simulink model "euler_equation"  (R2021b)
settings: Solver=VariableStepAuto  StartTime=0.0  StopTime=10.0  RelTol=1e-3
values from neighbouring files (symbols this model uses):
  J = [Ixx 0 0; 0 Iyy 0; 0 0 Izz]    [lab3_task1.m]    (also in lab3_task2.m; lab3_task3.m)
  Jinv = inv(J)    [lab3_task1.m]    (also in lab3_task2.m; lab3_task3.m)
  w0 = [0.45 0.52 0.55]'    [lab3_task1.m]    (also in lab3_task2.m; lab3_task3.m = w0_matrix(3,:)')
libraries: matrix_library x1
settings Model: Creator=samuz  LastModifiedBy=samuz

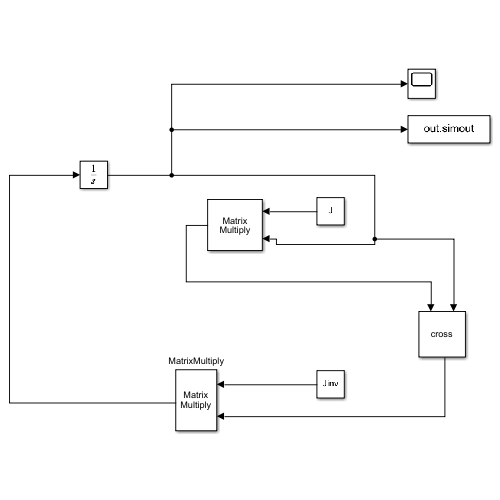
[thumbnail: Simulink's stored preview of the top-level diagram]
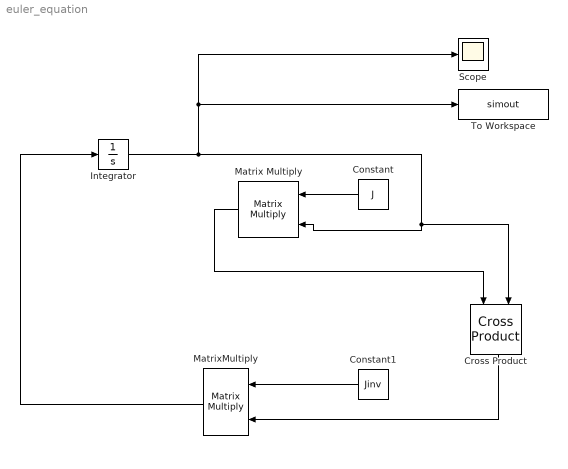
== system euler_equation ==
  Constant : Constant  Value=J
  Constant1 : Constant  Value=Jinv
  Cross Product : matrix_library/Cross Product
      settings: SourceProductBaseCode=SL
  Integrator : Integrator  InitialCondition=w0
  Matrix Multiply : Product  Multiplication=Matrix(*)
  MatrixMultiply : Product  Multiplication=Matrix(*)
  Scope : Scope
  To Workspace : ToWorkspace  VariableName=simout  SampleTime=-1
  wires:
  Matrix Multiply/1 -> Cross Product/1
  Cross Product/1 -> MatrixMultiply/2
  Integrator/1 -> Scope/1, To Workspace/1, Cross Product/2, Matrix Multiply/2
  Constant1/1 -> MatrixMultiply/1
  MatrixMultiply/1 -> Integrator/1
  Constant/1 -> Matrix Multiply/1
